simulink model "FCU"  (R2025b)
settings: Solver=VariableStepAuto  StartTime=0.0  StopTime=10.0  RelTol=1e-3
values from neighbouring files (symbols this model uses):
  I_max = 50    [Battery Trial.m]
  R_int = 0.1    [Battery Trial.m]
  V_min = 10    [Battery Trial.m]
  V_nom = 15    [Battery Trial.m]
undefined symbols (not defined in the file or in its folder): arm_lgt, C, Inertia, K_d, K_i, K_p, tau
libraries: simulink x7, vrlib x1
settings Model: Creator=zorb2  LastModifiedBy=zorb2

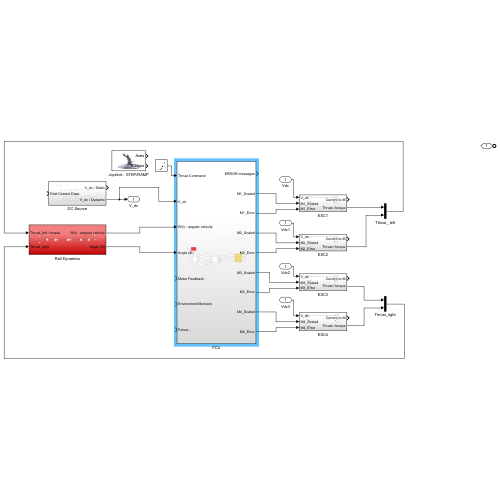
[thumbnail: Simulink's stored preview of the top-level diagram]
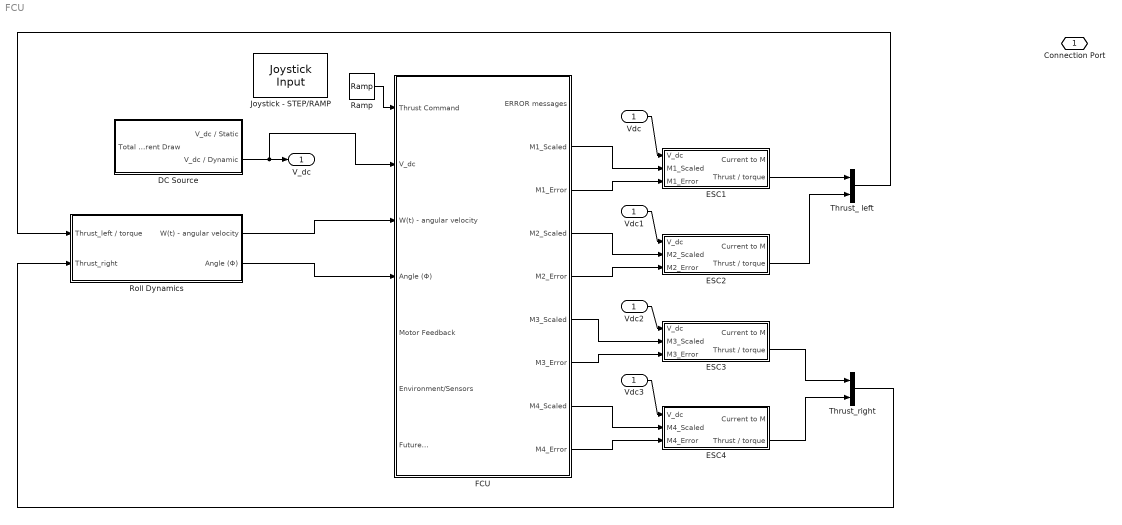
== system FCU ==
  Vdc : Inport
  DC Source : Subsystem
  ESC1 : Subsystem
  ESC2 : Subsystem
  ESC3 : Subsystem
  ESC4 : Subsystem
  FCU : Subsystem
  Joystick - STEP/RAMP : vrlib/Joystick Input  joyid=1  adjustports=on  forcefeed=off
  Ramp : simulink/Sources/Ramp  slope=0.5  start=0  InitialOutput=0
  Roll Dynamics : Subsystem
  Thrust_ left : Mux  Inputs=2
  Thrust_right : Mux  Inputs=2
  Vdc1 : InportShadow
  Vdc2 : InportShadow
  Vdc3 : InportShadow
  Connection Port : PMIOPort  Side=Left
  V_dc : Outport
  wires:
  FCU/2(M1_Scaled) -> ESC1/2(M1_Scaled)
  FCU/4(M2_Scaled) -> ESC2/2(M2_Scaled)
  FCU/6(M3_Scaled) -> ESC3/2(M3_Scaled)
  FCU/8(M4_Scaled) -> ESC4/2(M4_Scaled)
  FCU/9(M4_Error) -> ESC4/3(M4_Error)
  FCU/3(M1_Error) -> ESC1/3(M1_Error)
  FCU/5(M2_Error) -> ESC2/3(M2_Error)
  FCU/7(M3_Error) -> ESC3/3(M3_Error)
  Vdc/1 -> ESC1/1(V_dc)
  Vdc1/1 -> ESC2/1(V_dc)
  Vdc2/1 -> ESC3/1(V_dc)
  Vdc3/1 -> ESC4/1(V_dc)
  DC Source/2(V_dc / Dynamic) -> FCU/2(V_dc), V_dc/1
  Ramp/1 -> FCU/1(Thrust Command)
  Roll Dynamics/1(W(t) - angular velocity) -> FCU/3(W(t) - angular velocity)
  Roll Dynamics/2(Angle (Φ)) -> FCU/4(Angle (Φ))
  ESC1/2(Thrust / torque) -> Thrust_ left/1
  ESC2/2(Thrust / torque) -> Thrust_ left/2
  ESC3/2(Thrust / torque) -> Thrust_right/1
  ESC4/2(Thrust / torque) -> Thrust_right/2
  Thrust_right/1 -> Roll Dynamics/2(Thrust_right)
  Thrust_ left/1 -> Roll Dynamics/1(Thrust_left / torque)

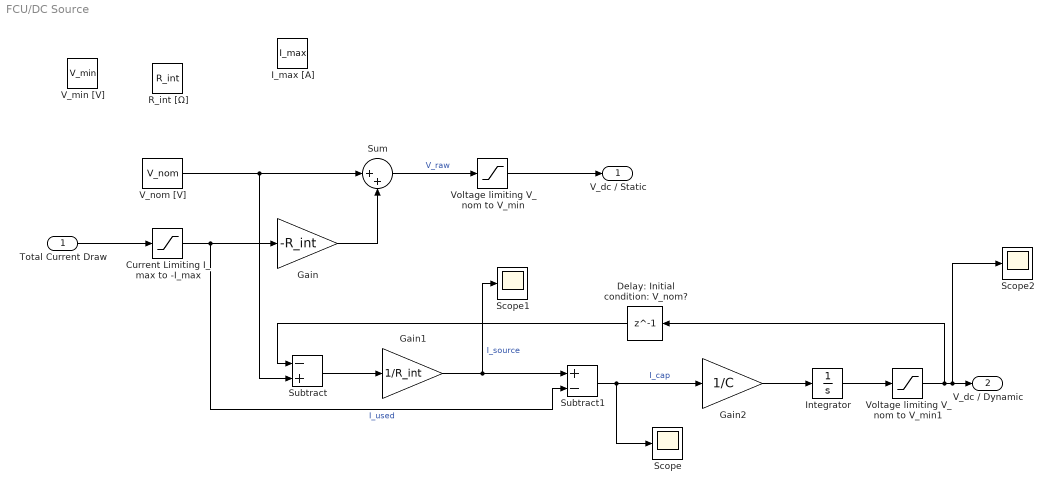
== system FCU/DC Source ==
  Total Current Draw : Inport
  Current Limiting I_max to -I_max : Saturate  UpperLimit=I_max  LowerLimit=-I_max
  Delay: Initial condition: V_nom? : Delay  DelayLength=1
  Gain : Gain  Gain=-R_int
  Gain1 : Gain  Gain=1/R_int
  Gain2 : Gain  Gain=1/C
  I_max [A] : Constant  Value=I_max
  Integrator : Integrator
  R_int [Ω] : Constant  Value=R_int
  Scope : Scope
  Scope1 : Scope
  Scope2 : Scope
      settings: DataLoggingVariableName=ScopeData2
  Subtract : Sum  Inputs=-+
  Subtract1 : Sum  Inputs=+-
  Sum : Sum  Inputs=|++
  V_min [V] : Constant  Value=V_min
  V_nom [V] : Constant  Value=V_nom
  Voltage limiting V_nom to V_min : Saturate  UpperLimit=V_nom  LowerLimit=V_min
  Voltage limiting V_nom to V_min1 : Saturate  UpperLimit=V_nom  LowerLimit=V_min
  V_dc / Static : Outport
  V_dc / Dynamic : Outport  Port=2
  wires:
  Current Limiting I_max to -I_max/1 -> Subtract1/2, Gain/1  "I_used"
  V_nom [V]/1 -> Sum/1, Subtract/2
  Gain/1 -> Sum/2
  Sum/1 -> Voltage limiting V_nom to V_min/1  "V_raw"
  Total Current Draw/1 -> Current Limiting I_max to -I_max/1
  Voltage limiting V_nom to V_min/1 -> V_dc / Static/1
  Subtract/1 -> Gain1/1
  Gain1/1 -> Scope1/1, Subtract1/1  "I_source"
  Subtract1/1 -> Scope/1, Gain2/1  "I_cap"
  Gain2/1 -> Integrator/1
  Integrator/1 -> Voltage limiting V_nom to V_min1/1
  Delay: Initial condition: V_nom?/1 -> Subtract/1
  Voltage limiting V_nom to V_min1/1 -> Delay: Initial condition: V_nom?/1, Scope2/1, V_dc / Dynamic/1

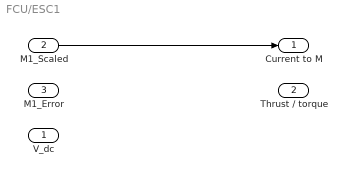
== system FCU/ESC1 ==
  V_dc : Inport
  M1_Scaled : Inport  Port=2
  M1_Error : Inport  Port=3
  Current to M : Outport
  Thrust / torque : Outport  Port=2
  wires:
  M1_Scaled/1 -> Current to M/1

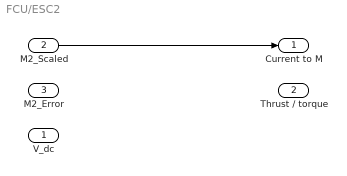
== system FCU/ESC2 ==
  V_dc : Inport
  M2_Scaled : Inport  Port=2
  M2_Error : Inport  Port=3
  Current to M : Outport
  Thrust / torque : Outport  Port=2
  wires:
  M2_Scaled/1 -> Current to M/1

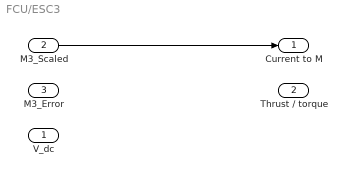
== system FCU/ESC3 ==
  V_dc : Inport
  M3_Scaled : Inport  Port=2
  M3_Error : Inport  Port=3
  Current to M : Outport
  Thrust / torque : Outport  Port=2
  wires:
  M3_Scaled/1 -> Current to M/1

== system FCU/ESC4 ==
  V_dc : Inport
  M4_Scaled : Inport  Port=2
  M4_Error : Inport  Port=3
  Current to M : Outport
  Thrust / torque : Outport  Port=2
  wires:
  M4_Scaled/1 -> Current to M/1

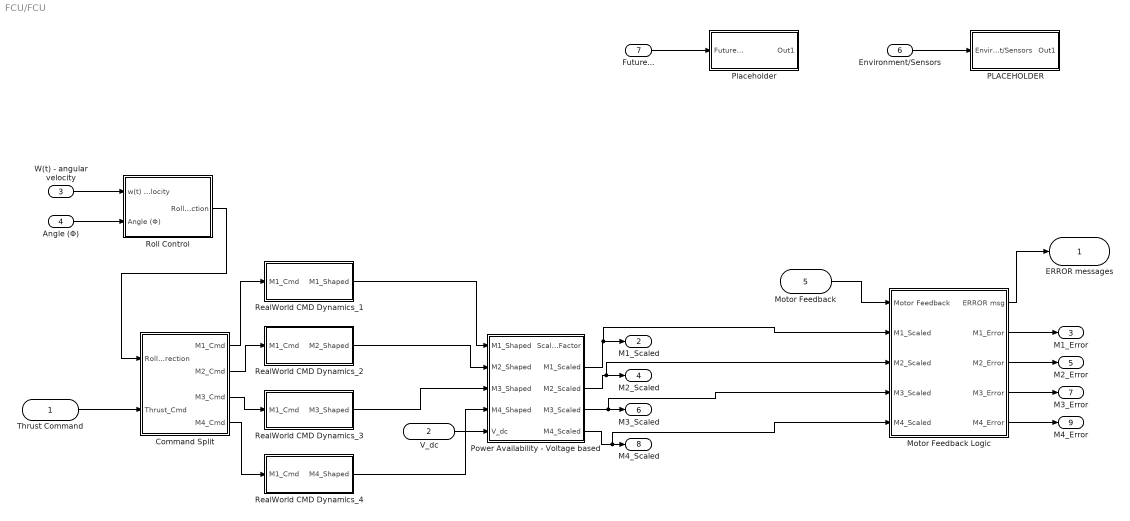
== system FCU/FCU ==
  Thrust Command : Inport
  V_dc : Inport  Port=2
  W(t) - angular velocity : Inport  Port=3
  Angle (Φ) : Inport  Port=4
  Motor Feedback : Inport  Port=5
  Environment/Sensors : Inport  Port=6
  Future... : Inport  Port=7
  Command Split : Subsystem
  Motor Feedback Logic : Subsystem
  PLACEHOLDER : Subsystem
  Placeholder : Subsystem
  Power Availability - Voltage based : Subsystem
  RealWorld CMD Dynamics_1 : Subsystem
  RealWorld CMD Dynamics_2 : Subsystem
  RealWorld CMD Dynamics_3 : Subsystem
  RealWorld CMD Dynamics_4 : Subsystem
  Roll Control : Subsystem
  ERROR messages : Outport
  M1_Scaled : Outport  Port=2
  M1_Error : Outport  Port=3
  M2_Scaled : Outport  Port=4
  M2_Error : Outport  Port=5
  M3_Scaled : Outport  Port=6
  M3_Error : Outport  Port=7
  M4_Scaled : Outport  Port=8
  M4_Error : Outport  Port=9
  wires:
  Thrust Command/1 -> Command Split/2(Thrust_Cmd)
  Command Split/1(M1_Cmd) -> RealWorld CMD Dynamics_1/1(M1_Cmd)
  Command Split/2(M2_Cmd) -> RealWorld CMD Dynamics_2/1(M1_Cmd)
  Command Split/3(M3_Cmd) -> RealWorld CMD Dynamics_3/1(M1_Cmd)
  Command Split/4(M4_Cmd) -> RealWorld CMD Dynamics_4/1(M1_Cmd)
  RealWorld CMD Dynamics_1/1(M1_Shaped) -> Power Availability - Voltage based/1(M1_Shaped)
  RealWorld CMD Dynamics_2/1(M2_Shaped) -> Power Availability - Voltage based/2(M2_Shaped)
  RealWorld CMD Dynamics_3/1(M3_Shaped) -> Power Availability - Voltage based/3(M3_Shaped)
  RealWorld CMD Dynamics_4/1(M4_Shaped) -> Power Availability - Voltage based/4(M4_Shaped)
  V_dc/1 -> Power Availability - Voltage based/5(V_dc)
  Power Availability - Voltage based/2(M1_Scaled) -> Motor Feedback Logic/2(M1_Scaled), M1_Scaled/1
  Power Availability - Voltage based/3(M2_Scaled) -> Motor Feedback Logic/3(M2_Scaled), M2_Scaled/1
  Power Availability - Voltage based/4(M3_Scaled) -> Motor Feedback Logic/4(M3_Scaled), M3_Scaled/1
  Power Availability - Voltage based/5(M4_Scaled) -> Motor Feedback Logic/5(M4_Scaled), M4_Scaled/1
  Motor Feedback/1 -> Motor Feedback Logic/1(Motor Feedback)
  Motor Feedback Logic/1(ERROR msg) -> ERROR messages/1
  Environment/Sensors/1 -> PLACEHOLDER/1(Environment/Sensors)
  Future.../1 -> Placeholder/1(Future...)
  Motor Feedback Logic/3(M2_Error) -> M2_Error/1
  Motor Feedback Logic/5(M4_Error) -> M4_Error/1
  Motor Feedback Logic/4(M3_Error) -> M3_Error/1
  Motor Feedback Logic/2(M1_Error) -> M1_Error/1
  W(t) - angular velocity/1 -> Roll Control/1(w(t) - angular velocity)
  Angle (Φ)/1 -> Roll Control/2(Angle (Φ))
  Roll Control/1(Roll_correction) -> Command Split/1(Roll_correction)

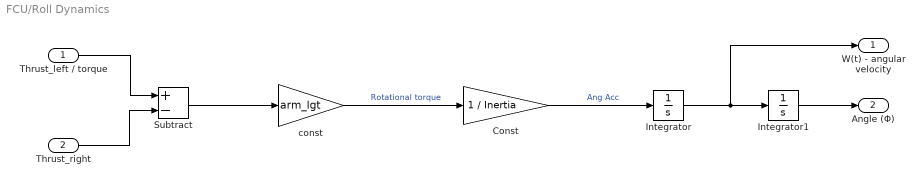
== system FCU/Roll Dynamics ==
  Thrust_left / torque : Inport
  Thrust_right : Inport  Port=2
  Const : Gain  Gain=1 / Inertia
  Integrator : Integrator
  Integrator1 : Integrator
  Subtract : Sum  Inputs=+-
  const : Gain  Gain=arm_lgt
  W(t) - angular velocity : Outport
  Angle (Φ) : Outport  Port=2
  wires:
  Thrust_left / torque/1 -> Subtract/1
  Thrust_right/1 -> Subtract/2
  Subtract/1 -> const/1
  const/1 -> Const/1  "Rotational torque"
  Const/1 -> Integrator/1  "Ang Acc"
  Integrator/1 -> Integrator1/1, W(t) - angular velocity/1
  Integrator1/1 -> Angle (Φ)/1

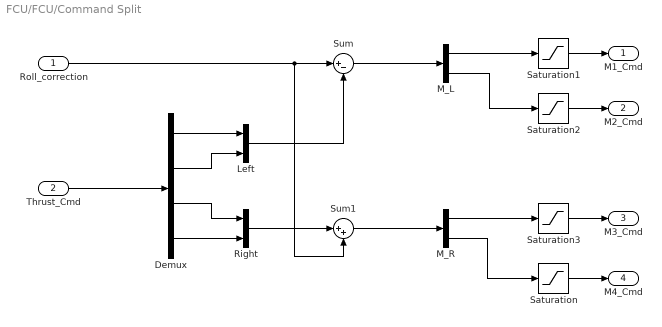
== system FCU/FCU/Command Split ==
  Roll_correction : Inport
  Thrust_Cmd : Inport  Port=2
  Demux : Demux
  Left : Mux  Inputs=2
  M_L : Demux  Outputs=2
  M_R : Demux  Outputs=2
  Right : Mux  Inputs=2
  Saturation{,1..3} (4 alike) : Saturate  UpperLimit=1  LowerLimit=0
  Sum : Sum  Inputs=|+-
  Sum1 : Sum  Inputs=|++
  M1_Cmd : Outport
  M2_Cmd : Outport  Port=2
  M3_Cmd : Outport  Port=3
  M4_Cmd : Outport  Port=4
  wires:
  Thrust_Cmd/1 -> Demux/1
  Demux/1 -> Left/1
  Demux/2 -> Left/2
  Demux/4 -> Right/2
  Demux/3 -> Right/1
  Left/1 -> Sum/2
  Right/1 -> Sum1/1
  Roll_correction/1 -> Sum1/2, Sum/1
  Sum/1 -> M_L/1
  Sum1/1 -> M_R/1
  M_L/1 -> Saturation1/1
  M_L/2 -> Saturation2/1
  M_R/1 -> Saturation3/1
  M_R/2 -> Saturation/1
  Saturation1/1 -> M1_Cmd/1
  Saturation2/1 -> M2_Cmd/1
  Saturation3/1 -> M3_Cmd/1
  Saturation/1 -> M4_Cmd/1

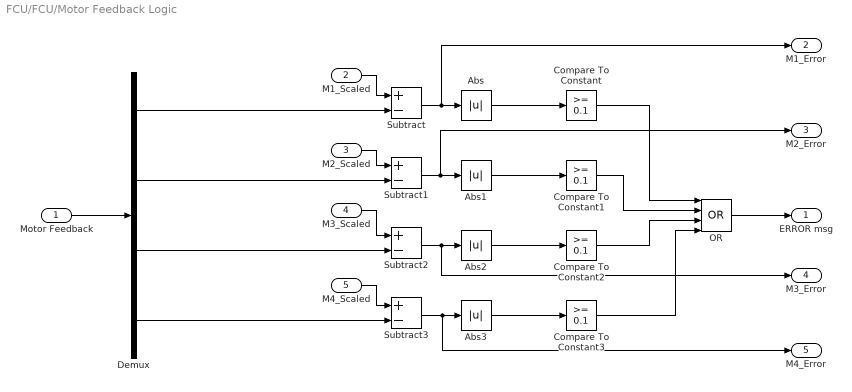
== system FCU/FCU/Motor Feedback Logic ==
  Motor Feedback : Inport
  M1_Scaled : Inport  Port=2
  M2_Scaled : Inport  Port=3
  M3_Scaled : Inport  Port=4
  M4_Scaled : Inport  Port=5
  Abs{,1..3} (4 alike) : Abs  SaturateOnIntegerOverflow=off
  Compare To Constant{,1..3} (4 alike) : simulink/Logic and Bit Operations/Compare To Constant  relop=>=  const=0.1  OutDataTypeStr=boolean
  Demux : Demux
  OR : Logic  Operator=OR  Inputs=4  IconShape=distinctive  AllPortsSameDT=off  OutDataTypeStr=boolean
  Subtract{,1..3} (4 alike) : Sum  Inputs=+-
  ERROR msg : Outport
  M1_Error : Outport  Port=2
  M2_Error : Outport  Port=3
  M3_Error : Outport  Port=4
  M4_Error : Outport  Port=5
  wires:
  Motor Feedback/1 -> Demux/1
  Demux/1 -> Subtract/2
  Demux/2 -> Subtract1/2
  Demux/4 -> Subtract3/2
  Subtract/1 -> M1_Error/1, Abs/1
  Subtract1/1 -> M2_Error/1, Abs1/1
  Subtract2/1 -> M3_Error/1, Abs2/1
  Subtract3/1 -> M4_Error/1, Abs3/1
  Demux/3 -> Subtract2/2
  Abs/1 -> Compare To Constant/1
  Abs3/1 -> Compare To Constant3/1
  Abs2/1 -> Compare To Constant2/1
  Abs1/1 -> Compare To Constant1/1
  Compare To Constant/1 -> OR/1
  Compare To Constant1/1 -> OR/2
  Compare To Constant2/1 -> OR/3
  Compare To Constant3/1 -> OR/4
  OR/1 -> ERROR msg/1
  M1_Scaled/1 -> Subtract/1
  M2_Scaled/1 -> Subtract1/1
  M3_Scaled/1 -> Subtract2/1
  M4_Scaled/1 -> Subtract3/1

== system FCU/FCU/PLACEHOLDER ==
  Environment/Sensors : Inport
  Out1 : Outport
  wires:
  Environment/Sensors/1 -> Out1/1

== system FCU/FCU/Placeholder ==
  Future... : Inport
  Out1 : Outport
  wires:
  Future.../1 -> Out1/1

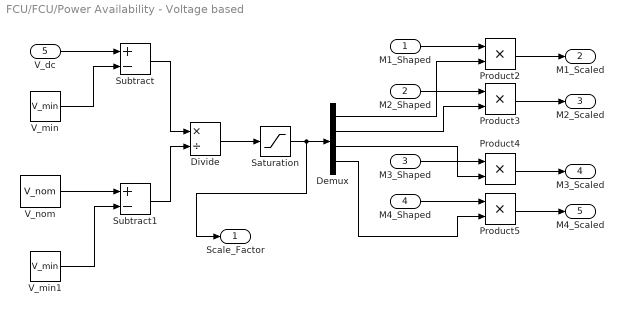
== system FCU/FCU/Power Availability - Voltage based ==
  M1_Shaped : Inport
  M2_Shaped : Inport  Port=2
  M3_Shaped : Inport  Port=3
  M4_Shaped : Inport  Port=4
  V_dc : Inport  Port=5
  Demux : Demux
  Divide : Product  Inputs=*/
  Product{2..5} (4 alike) : Product
  Saturation : Saturate  UpperLimit=1  LowerLimit=0
  Subtract : Sum  Inputs=+-
  Subtract1 : Sum  Inputs=+-
  V_min : Constant  Value=V_min
  V_min1 : Constant  Value=V_min
  V_nom : Constant  Value=V_nom
  Scale_Factor : Outport
  M1_Scaled : Outport  Port=2
  M2_Scaled : Outport  Port=3
  M3_Scaled : Outport  Port=4
  M4_Scaled : Outport  Port=5
  wires:
  V_dc/1 -> Subtract/1
  V_min/1 -> Subtract/2
  V_min1/1 -> Subtract1/2
  V_nom/1 -> Subtract1/1
  Subtract/1 -> Divide/1
  Divide/1 -> Saturation/1
  M1_Shaped/1 -> Product2/1
  M2_Shaped/1 -> Product3/1
  M3_Shaped/1 -> Product4/1
  M4_Shaped/1 -> Product5/1
  Saturation/1 -> Scale_Factor/1, Demux/1
  Demux/1 -> Product2/2
  Demux/2 -> Product3/2
  Demux/3 -> Product4/2
  Demux/4 -> Product5/2
  Subtract1/1 -> Divide/2
  Product2/1 -> M1_Scaled/1
  Product3/1 -> M2_Scaled/1
  Product4/1 -> M3_Scaled/1
  Product5/1 -> M4_Scaled/1

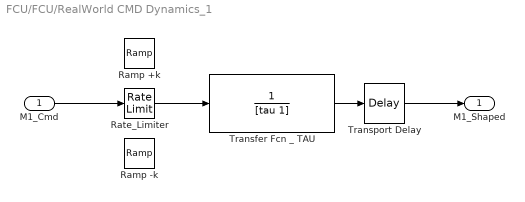
== system FCU/FCU/RealWorld CMD Dynamics_1 ==
  M1_Cmd : Inport
  Ramp +k : simulink/Sources/Ramp  slope=1  start=0  InitialOutput=0
  Ramp -k : simulink/Sources/Ramp  slope=1  start=0  InitialOutput=0
  Rate_Limiter : RateLimiter  SampleTimeMode=inherited
  Transfer Fcn _ TAU : TransferFcn  Denominator=[tau 1]
  Transport Delay : TransportDelay
  M1_Shaped : Outport
  wires:
  M1_Cmd/1 -> Rate_Limiter/1
  Rate_Limiter/1 -> Transfer Fcn _ TAU/1
  Transfer Fcn _ TAU/1 -> Transport Delay/1
  Transport Delay/1 -> M1_Shaped/1

== system FCU/FCU/RealWorld CMD Dynamics_2 ==
  M1_Cmd : Inport
  Rate Limiter : RateLimiter  SampleTimeMode=inherited
  Transfer Fcn_TAU : TransferFcn  Denominator=[1 1]
  Transport Delay : TransportDelay
  M2_Shaped : Outport
  wires:
  Transport Delay/1 -> M2_Shaped/1
  Transfer Fcn_TAU/1 -> Transport Delay/1
  Rate Limiter/1 -> Transfer Fcn_TAU/1
  M1_Cmd/1 -> Rate Limiter/1

== system FCU/FCU/RealWorld CMD Dynamics_3 ==
  M1_Cmd : Inport
  Rate Limiter : RateLimiter  SampleTimeMode=inherited
  Transfer Fcn_TAU : TransferFcn  Denominator=[1 1]
  Transport Delay : TransportDelay
  M3_Shaped : Outport
  wires:
  M1_Cmd/1 -> Rate Limiter/1
  Rate Limiter/1 -> Transfer Fcn_TAU/1
  Transfer Fcn_TAU/1 -> Transport Delay/1
  Transport Delay/1 -> M3_Shaped/1

== system FCU/FCU/RealWorld CMD Dynamics_4 ==
  M1_Cmd : Inport
  Rate Limiter : RateLimiter  SampleTimeMode=inherited
  Transfer Fcn_TAU : TransferFcn  Denominator=[1 1]
  Transport Delay : TransportDelay
  M4_Shaped : Outport
  wires:
  Transport Delay/1 -> M4_Shaped/1
  Transfer Fcn_TAU/1 -> Transport Delay/1
  Rate Limiter/1 -> Transfer Fcn_TAU/1
  M1_Cmd/1 -> Rate Limiter/1

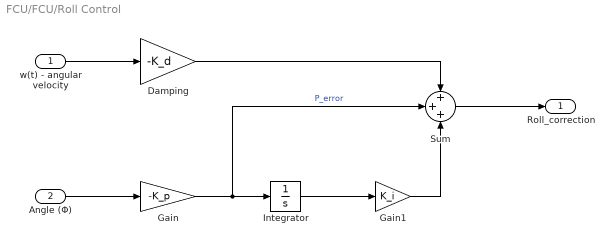
== system FCU/FCU/Roll Control ==
  w(t) - angular velocity : Inport
  Angle (Φ) : Inport  Port=2
  Damping : Gain  Gain=-K_d
  Gain : Gain  Gain=-K_p
  Gain1 : Gain  Gain=K_i
  Integrator : Integrator
  Sum : Sum  Inputs=+++
  Roll_correction : Outport
  wires:
  Angle (Φ)/1 -> Gain/1
  Gain/1 -> Sum/2, Integrator/1  "P_error"
  w(t) - angular velocity/1 -> Damping/1
  Integrator/1 -> Gain1/1
  Damping/1 -> Sum/1
  Gain1/1 -> Sum/3
  Sum/1 -> Roll_correction/1
